simulink library "leastSquaresSolution_ul"  (R2018a)
settings: Solver=VariableStepAuto  StartTime=0.0  StopTime=10.0  RelTol=1e-3
settings Model: Creator=mitch  LastModifiedBy=mitch

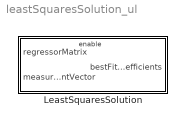
== system leastSquaresSolution_ul ==
  LeastSquaresSolution : Subsystem

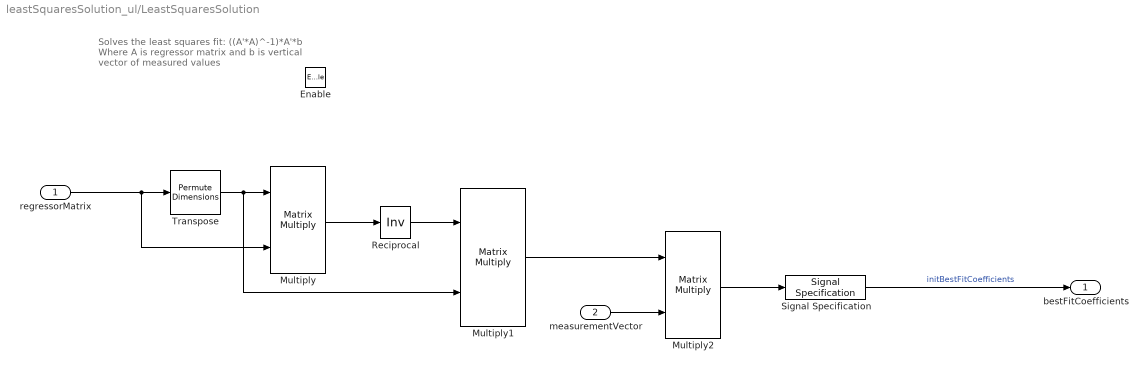
== system leastSquaresSolution_ul/LeastSquaresSolution ==
  note: Solves the least squares fit:
      | ((A'*A)^-1)*A'*b
      | Where A is regressor matrix
      | and b is vertical vector of measured values
  regressorMatrix : Inport
  measurementVector : Inport  Port=2
  Enable : EnablePort
  Multiply : Product  Multiplication=Matrix(*)
  Multiply1 : Product  Multiplication=Matrix(*)
  Multiply2 : Product  Multiplication=Matrix(*)
  Reciprocal : Product  Inputs=/  Multiplication=Matrix(*)
  Signal Specification : SignalSpecification  Dimensions=[5 1]
  Transpose : PermuteDimensions
  bestFitCoefficients : Outport
  wires:
  Multiply/1 -> Reciprocal/1
  regressorMatrix/1 -> Multiply/2, Transpose/1
  Transpose/1 -> Multiply1/2, Multiply/1
  measurementVector/1 -> Multiply2/2
  Multiply2/1 -> Signal Specification/1
  Reciprocal/1 -> Multiply1/1
  Multiply1/1 -> Multiply2/1
  Signal Specification/1 -> bestFitCoefficients/1  "initBestFitCoefficients"
